simulink model "Model"  (R2015b)
settings: Solver=VariableStepAuto  StartTime=0.0  StopTime=2  RelTol=1e-3
libraries: truetime x10
settings Model: Creator=USUARIO  LastModifiedBy=USUARIO

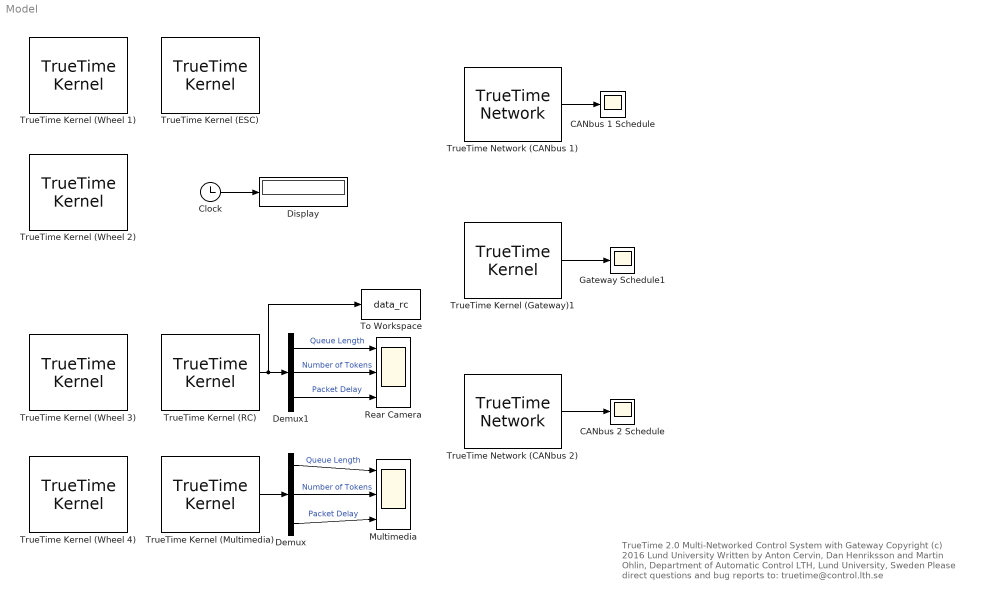
== system Model ==
  note: TrueTime 2.0  Multi-Networked Control System with Gateway
      | Copyright (c) 2016 Lund University
      | Written by Anton Cervin, Dan Henriksson and Martin Ohlin,
      | Department of Automatic Control LTH, Lund University, Sweden
      | Please direct questions and bug reports to:  truetime@control.lth.se
  CANbus 1 Schedule : Scope
  CANbus 2 Schedule : Scope
  Clock : Clock
  Demux : Demux  Outputs=3
  Demux1 : Demux  Outputs=3
  Display : Display
  Gateway Schedule1 : Scope
  Multimedia : Scope  NumInputPorts=3
  Rear Camera : Scope  NumInputPorts=3
  To Workspace : ToWorkspace  VariableName=data_rc  SaveFormat=Timeseries  SampleTime=-1
  TrueTime Kernel (ESC) : truetime/TrueTime Kernel  Priority=1  sfun=esc_init  args=[]  ninputsoutputs=[0 0]  ntriggers=0  trigtype=rising  nwnodenbr=[1 2]  clockoffsetdrift=[0 0]  schedoutput=off  battery=off  poweroutput=off  label=1: 2
  TrueTime Kernel (Gateway)1 : truetime/TrueTime Kernel  Priority=1  sfun=gateway_init  args=[]  ninputsoutputs=[0 0]  ntriggers=0  trigtype=rising  nwnodenbr=[1 1;2 1]  clockoffsetdrift=[0 0]  schedoutput=on  battery=off  poweroutput=off  label=1: 1\n2: 1
  TrueTime Kernel (Multimedia) : truetime/TrueTime Kernel  Priority=1  sfun=multimedia_init  args=[]  ninputsoutputs=[0 3]  ntriggers=0  trigtype=rising  nwnodenbr=[2 5]  clockoffsetdrift=[0 0]  schedoutput=off  battery=off  poweroutput=off  label=2: 5
  TrueTime Kernel (RC) : truetime/TrueTime Kernel  Priority=1  sfun=rc_init  args=[]  ninputsoutputs=[0 3]  ntriggers=0  trigtype=rising  nwnodenbr=[2 3]  clockoffsetdrift=[0 0]  schedoutput=off  battery=off  poweroutput=off  label=2: 3
  TrueTime Kernel (Wheel 1) : truetime/TrueTime Kernel  Priority=1  sfun=wheel_init  args=[]  ninputsoutputs=[0 0]  ntriggers=0  trigtype=rising  nwnodenbr=[1 3]  clockoffsetdrift=[0 0]  schedoutput=off  battery=off  poweroutput=off  label=1: 3
  TrueTime Kernel (Wheel 2) : truetime/TrueTime Kernel  Priority=1  sfun=wheel_init  args=[]  ninputsoutputs=[0 0]  ntriggers=0  trigtype=rising  nwnodenbr=[1 6]  clockoffsetdrift=[0 0]  schedoutput=off  battery=off  poweroutput=off  label=1: 6
  TrueTime Kernel (Wheel 3) : truetime/TrueTime Kernel  Priority=1  sfun=wheel_init  args=[]  ninputsoutputs=[0 0]  ntriggers=0  trigtype=rising  nwnodenbr=[2 2]  clockoffsetdrift=[0 0]  schedoutput=off  battery=off  poweroutput=off  label=2: 2
  TrueTime Kernel (Wheel 4) : truetime/TrueTime Kernel  Priority=1  sfun=wheel_init  args=[]  ninputsoutputs=[0 0]  ntriggers=0  trigtype=rising  nwnodenbr=[2 4]  clockoffsetdrift=[0 0]  schedoutput=off  battery=off  poweroutput=off  label=2: 4
  TrueTime Network (CANbus 1) : truetime/TrueTime Network  Priority=1  nwtype=CSMA/AMP (CAN)  nwnbr=1  nnodes=6  rate=1e6  minsize=29  lossprob=0  seed=0  bandwidths=[0.5 0.25 0.25]  slotsize=80  schedule=[1 2 1 3]  memsize=80000  buftype=Common buffer  overflow=Retransmit  dynSchedule=[]  miniSlotSize=40  NIT=0  QSortMode=FIFO  sync=0  irtSchedule=0  nrtLength=0  nodeGraph=0  scheduleoutput=on
  TrueTime Network (CANbus 2) : truetime/TrueTime Network  Priority=1  nwtype=CSMA/AMP (CAN)  nwnbr=2  nnodes=5  rate=1e6  minsize=29  lossprob=0  seed=0  bandwidths=[0.5 0.25 0.25]  slotsize=80  schedule=[1 2 1 3]  memsize=80000  buftype=Common buffer  overflow=Retransmit  dynSchedule=[]  miniSlotSize=40  NIT=0  QSortMode=FIFO  sync=0  irtSchedule=0  nrtLength=0  nodeGraph=0  scheduleoutput=on
  wires:
  Clock/1 -> Display/1
  TrueTime Network (CANbus 1)/1 -> CANbus 1 Schedule/1
  TrueTime Network (CANbus 2)/1 -> CANbus 2 Schedule/1
  TrueTime Kernel (Gateway)1/1 -> Gateway Schedule1/1
  TrueTime Kernel (Multimedia)/1 -> Demux/1
  Demux/1 -> Multimedia/1  "Queue Length"
  Demux/2 -> Multimedia/2  "Number of Tokens"
  Demux/3 -> Multimedia/3  "Packet Delay"
  TrueTime Kernel (RC)/1 -> To Workspace/1, Demux1/1
  Demux1/1 -> Rear Camera/1  "Queue Length"
  Demux1/2 -> Rear Camera/2  "Number of Tokens"
  Demux1/3 -> Rear Camera/3  "Packet Delay"
